simulink model "inverting"  (R2020b)
settings: Solver=VariableStepAuto  StartTime=0.0  StopTime=0.2  MaxStep=0.00002  RelTol=1e-3  AbsTol=1e-3  EnableMultiTasking=on
libraries: fl_lib x9, nesl_utility x3
CloseFcn:
  | try,close(h1_ssc_opamp_inverting),end
  | clear simlog_ssc_opamp_inverting
Description:
  | Op-Amp Circuit - Inverting Amplifier
settings Model: Creator=The MathWorks, Inc.  LastModifiedBy=bolic
settings SolverCC: AutoScaleAbsTol=off
settings DataIOCC: LimitDataPoints=on  SaveFormat=Array  ReturnWorkspaceOutputs=off
settings OptimizationCC: LifeSpan=inf
settings DebuggingCC: SolverPrmCheckMsg=warning  AllowSymbolicDim=off  PregeneratedLibrarySubsystemCodeDiagnostic=none  SFUnexpectedBacktrackingDiag=warning  SFNoUnconditionalDefaultTransitionDiag=warning  SFExecutionAtInitializationDiag=none  ArithmeticOperatorsInVariantConditions=warning
settings HardwareCC: ProdBitPerPointer=32  ProdBitPerSizeT=32  ProdBitPerPtrDiffT=32  ProdLargestAtomicFloat=None  ProdIntDivRoundTo=Undefined  ProdEndianess=Unspecified  ProdWordSize=32  ProdHWDeviceType=32-bit Generic
settings ModelReferenceCC: PropagateSignalLabelsOutOfModel=off
settings SFSimCC: SimUseLocalCustomCode=off  CustomCodeUndefinedFunction=UseInterfaceOnly
settings RTWCC: RTWUseLocalCustomCode=off
settings CodeAppCC: StateflowObjectComments=on
settings GRTTargetCC: TargetLangStandard=C89/C90 (ANSI)
settings ConfigComp: CovMetricSettings=dw  CovSaveCumulativeToWorkspaceVar=on  CovSaveSingleToWorkspaceVar=on  CovExternalEMLEnable=off  CovSFcnEnable=off
settings SimscapeCC: SimscapeLogType=all  SimscapeLogSimulationStatistics=on  SimscapeLogName=simlog_ssc_opamp_inverting  SimscapeLogDataHistory=10000

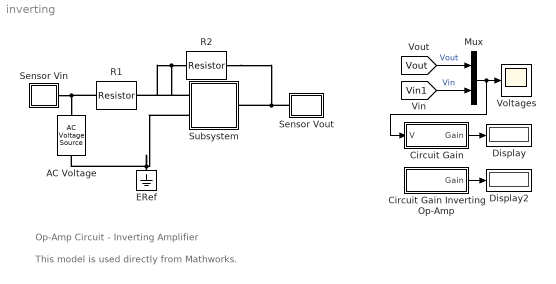
== system inverting ==
  note: This model is used directly from Mathworks.
  note: Op-Amp Circuit - Inverting Amplifier
  AC Voltage : fl_lib/Electrical/Electrical Sources/AC Voltage Source  amp=0.1 V  shift=0 deg  frequency=10 Hz  omega=0 rad/s
      settings: SourceProductName=Foundation Library
  Circuit Gain : Subsystem
  Circuit Gain Inverting Op-Amp : Subsystem
      mask init:
      | set_param([gcb '/R1'],'Value',...
      |     get_param([bdroot '/R1'],'r'));
      | set_param([gcb '/R2'],'Value',...
      |     get_param([bdroot '/R2'],'r'));
      mask Display: disp('-R2/R1')
  Display : Display
  Display2 : Display
  ERef : fl_lib/Electrical/Electrical Elements/Electrical Reference
      settings: SourceProductName=Foundation Library
  Mux : Mux  Inputs=2
  R1 : fl_lib/Electrical/Electrical Elements/Resistor  R=1 kOhm  i_specify=off  i_priority=High  i=0 A  i_nominal_specify=off  i_nominal_unit=A  i_nominal_value=1  v_specify=off  v_priority=High  v=0 V  v_nominal_specify=off  v_nominal_unit=V  v_nominal_value=1
      settings: AttributesFormatString=%<R> %<R_unit>  SourceProductName=Foundation Library
  R2 : fl_lib/Electrical/Electrical Elements/Resistor  R=10 kOhm  i_specify=off  i_priority=High  i=0 A  i_nominal_specify=off  i_nominal_unit=A  i_nominal_value=1  v_specify=off  v_priority=High  v=0 V  v_nominal_specify=off  v_nominal_unit=V  v_nominal_value=1
      settings: AttributesFormatString=%<R> %<R_unit>  SourceProductName=Foundation Library
  Sensor Vin : Subsystem
      mask Display: disp('Vin')
  Sensor Vout : Subsystem
      mask Display: disp('Vo')
  Subsystem : Subsystem
      mask Display: image('op_amp.png')
  Voltages : Scope
  wires:
  Mux/1 -> Circuit Gain/1(V), Voltages/1
  [Vout] -> Mux/1  "Vout"
  [Vin1] -> Mux/2  "Vin"
  Circuit Gain/1(Gain) -> Display/1
  Circuit Gain Inverting Op-Amp/1(Gain) -> Display2/1
  connections:
  ERef/LConn1 -- Subsystem/LConn2 -- AC Voltage/RConn1
  R1/LConn1 -- Sensor Vin/LConn1 -- AC Voltage/LConn1
  R2/RConn1 -- Sensor Vout/LConn1 -- Subsystem/RConn1
  R2/LConn1 -- Subsystem/LConn1 -- R1/RConn1

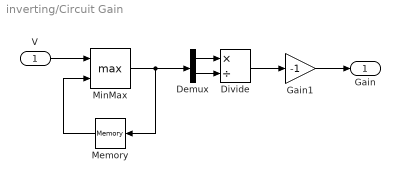
== system inverting/Circuit Gain ==
  V : Inport
  Demux : Demux  Outputs=2
  Divide : Product  Inputs=*/
  Gain1 : Gain  Gain=-1
  Memory : Memory  InitialCondition=1e-15  InheritSampleTime=on
  MinMax : MinMax  DisableCoverage=on  Function=max  Inputs=2  OutDataTypeStr=Inherit: Inherit via back propagation  ZeroCross=off
      settings: LockScale=on
  Gain : Outport  VectorParamsAs1DForOutWhenUnconnected=off
  wires:
  Gain1/1 -> Gain/1
  Divide/1 -> Gain1/1
  Demux/2 -> Divide/2
  Memory/1 -> MinMax/2
  MinMax/1 -> Demux/1, Memory/1
  Demux/1 -> Divide/1
  V/1 -> MinMax/1

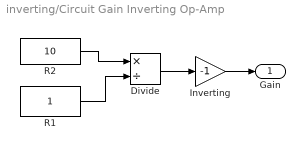
== system inverting/Circuit Gain Inverting Op-Amp ==
  Divide : Product  Inputs=*/
  Inverting : Gain  Gain=-1
  R1 : Constant
  R2 : Constant  Value=10
  Gain : Outport  VectorParamsAs1DForOutWhenUnconnected=off
  wires:
  R2/1 -> Divide/1
  R1/1 -> Divide/2
  Inverting/1 -> Gain/1
  Divide/1 -> Inverting/1

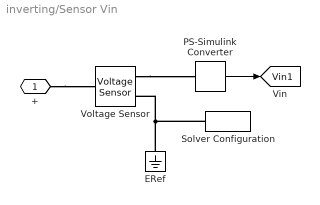
== system inverting/Sensor Vin ==
  ERef : fl_lib/Electrical/Electrical Elements/Electrical Reference
      settings: SourceProductName=Foundation Library
  PS-Simulink Converter : nesl_utility/PS-Simulink Converter  PhysicalDomain=network_engine_domain  SubClassName=ps_output  LeftPortType=input  RightPortType=output  PseudoPeriodic=off  Frequencies=[]  Unit=1  AffineConversion=off
      settings: SourceProductName=Utilities
  Solver Configuration : nesl_utility/Solver Configuration  PhysicalDomain=network_engine_domain  SubClassName=solver  LeftPortType=input  RightPortType=generic  Tones=[]  Harmonics=[]  SimulateNoise=off  Profile=off  UseLocalSampling=off  EnableSwitchedLinearOptims=on  FrequencyDomain=off  UseCCode=off  RelTol=0.001  AbsTol=1e-06  MinStep=1e-09  ToWorkspace=off  RevertToSquareIcSolve=off  NumHomotopyIterations=100  PhasorMode=off  PhasorModeNumHarmonics=1  DoDC=off  ResidualTolerance=1e-9  UseLocalSolver=off  LocalSolverChoice=NE_BACKWARD_EULER_ADVANCER  LocalSolverSampleTime=1e-6  DoFixedCost=off  MaxNonlinIter=3  MaxModeIter=2  ComputeImpulses=off  ImpulseIterations=2  LinearAlgebra=auto  EquationFormulation=NE_TIME_EF  DelaysMemoryBudget=1024  AutomaticFiltering=on  FilteringTimeConstant=0.001  PartitionStorageMethod=AS_NEEDED  PartitionMemoryBudget=1024  PartitionMethod=FAST
      settings: SourceProductName=Utilities
  Voltage Sensor : fl_lib/Electrical/Electrical Sensors/Voltage Sensor
      settings: SourceProductName=Foundation Library
  + : PMIOPort  Side=Left
  tag scope: Vin1=global
  wires:
  PS-Simulink Converter/1 -> [Vin1]
  connections:
  +/RConn1 -- Voltage Sensor/LConn1
  Voltage Sensor/RConn1 -- PS-Simulink Converter/LConn1
  ERef/LConn1 -- Solver Configuration/RConn1 -- Voltage Sensor/RConn2

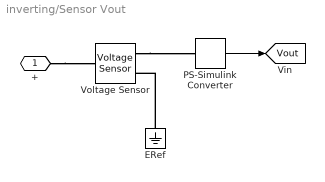
== system inverting/Sensor Vout ==
  ERef : fl_lib/Electrical/Electrical Elements/Electrical Reference
      settings: SourceProductName=Foundation Library
  PS-Simulink Converter : nesl_utility/PS-Simulink Converter  PhysicalDomain=network_engine_domain  SubClassName=ps_output  LeftPortType=input  RightPortType=output  PseudoPeriodic=off  Frequencies=[]  Unit=1  AffineConversion=off
      settings: SourceProductName=Utilities
  Voltage Sensor : fl_lib/Electrical/Electrical Sensors/Voltage Sensor
      settings: SourceProductName=Foundation Library
  + : PMIOPort  Side=Left
  tag scope: Vout=global
  wires:
  PS-Simulink Converter/1 -> [Vout]
  connections:
  ERef/LConn1 -- Voltage Sensor/RConn2
  Voltage Sensor/RConn1 -- PS-Simulink Converter/LConn1
  +/RConn1 -- Voltage Sensor/LConn1

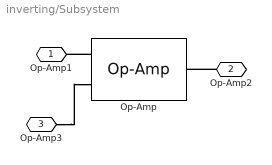
== system inverting/Subsystem ==
  Op-Amp : fl_lib/Electrical/Electrical Elements/Op-Amp  outI_specify=off  outI_priority=High  outI=0 A  outI_nominal_specify=off  outI_nominal_unit=A  outI_nominal_value=1
      settings: SourceProductName=Foundation Library
  Op-Amp1 : PMIOPort  Side=Left
  Op-Amp2 : PMIOPort  Port=2  Side=Right
  Op-Amp3 : PMIOPort  Port=3  Side=Left
  connections:
  Op-Amp3/RConn1 -- Op-Amp/LConn1
  Op-Amp2/RConn1 -- Op-Amp/RConn1
  Op-Amp/LConn2 -- Op-Amp1/RConn1
